simulink model "week2_3"  (R2020b)
settings: Solver=VariableStepAuto  StartTime=0.0  StopTime=10.0  RelTol=1e-3
model workspace (MAT data in the model file):
  M = Simulink.Parameter
  M.Value = 100
  M.DataType = 'auto'
  M.Dimensions = [1 1]
  b = Simulink.Parameter
  b.Value = 50
  b.DataType = 'auto'
  b.Dimensions = [1 1]
settings Model: Creator=Lenovo  LastModifiedBy=Lenovo

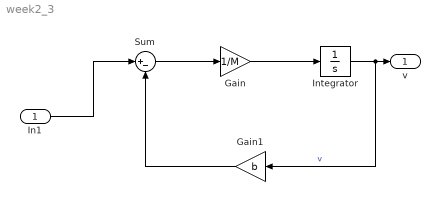
== system week2_3 ==
  In1 : Inport
  Gain : Gain  Gain=1/M
  Gain1 : Gain  Gain=b
  Integrator : Integrator
  Sum : Sum  Inputs=|+-
  v : Outport
  wires:
  Gain/1 -> Integrator/1
  Sum/1 -> Gain/1
  Gain1/1 -> Sum/2
  Integrator/1 -> Gain1/1, v/1  "v"
  In1/1 -> Sum/1
